simulink model "ODU_zad2"  (Simulink 6.3)
settings: Solver=ode45  StartTime=0.0  StopTime=0.6  RelTol=1e-3
settings Model: LastModifiedBy=Ms1

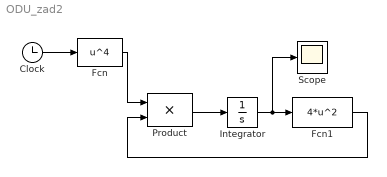
== system ODU_zad2 ==
  Clock : Clock
      settings: Decimation=10
  Fcn : Fcn  Expr=u^4
  Fcn1 : Fcn  Expr=4*u^2
  Integrator : Integrator  InitialCondition=10
  Product : Product  SaturateOnIntegerOverflow=on  InputSameDT=on
  Scope : Scope
  wires:
  Product/1 -> Integrator/1
  Clock/1 -> Fcn/1
  Integrator/1 -> Fcn1/1, Scope/1
  Fcn/1 -> Product/1
  Fcn1/1 -> Product/2
